simulink subsystem "ObOnePoleLpf"  (R2024a)
settings: Solver=VariableStepAuto  StartTime=0.0  StopTime=10.0  RelTol=1e-3
settings Model: Creator=dfurodet  LastModifiedBy=dfurodet

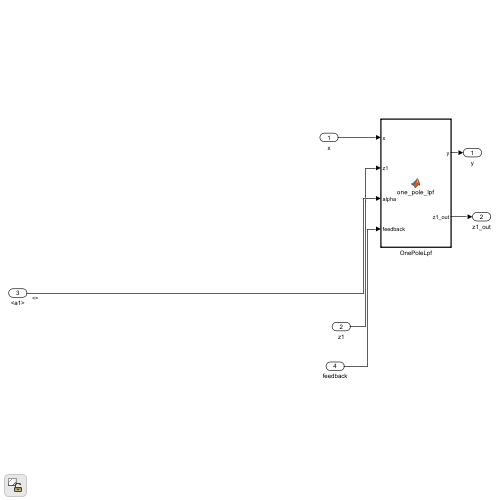
[thumbnail: Simulink's stored preview of the top-level diagram]
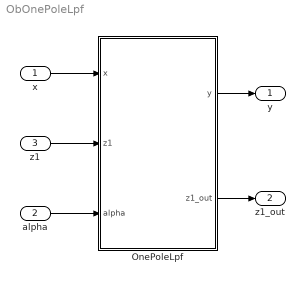
== system ObOnePoleLpf ==
  x : Inport
  alpha : Inport  Port=2
  z1 : Inport  Port=3  OutDataTypeStr=single
  OnePoleLpf : MATLAB Function  TreatAsAtomicUnit=on
  y : Outport
  z1_out : Outport  Port=2
  wires:
  alpha/1 -> OnePoleLpf/3(alpha)
  x/1 -> OnePoleLpf/1(x)
  OnePoleLpf/2(z1_out) -> z1_out/1
  z1/1 -> OnePoleLpf/2(z1)
  OnePoleLpf/1(y) -> y/1

== matlab function ObOnePoleLpf/OnePoleLpf ==
  data: x input; y output; z1 input; alpha input; z1_out output
function [y , z1_out] = one_pole_lpf(x, z1, alpha)
    feedback = 0;
    s = x + feedback;
    %feedback_output = beta * z1;
    vn = (s - z1) * alpha;
    y = vn + z1;
    z1_out = single(vn + y);
end
